simulink subsystem "ESD"  (R2020b)
settings: Solver=VariableStepAuto  StartTime=0.0  StopTime=10.0  RelTol=1e-3
undefined symbols (not defined in the file or in its folder): params
settings Model: Creator=trevor  LastModifiedBy=trevor

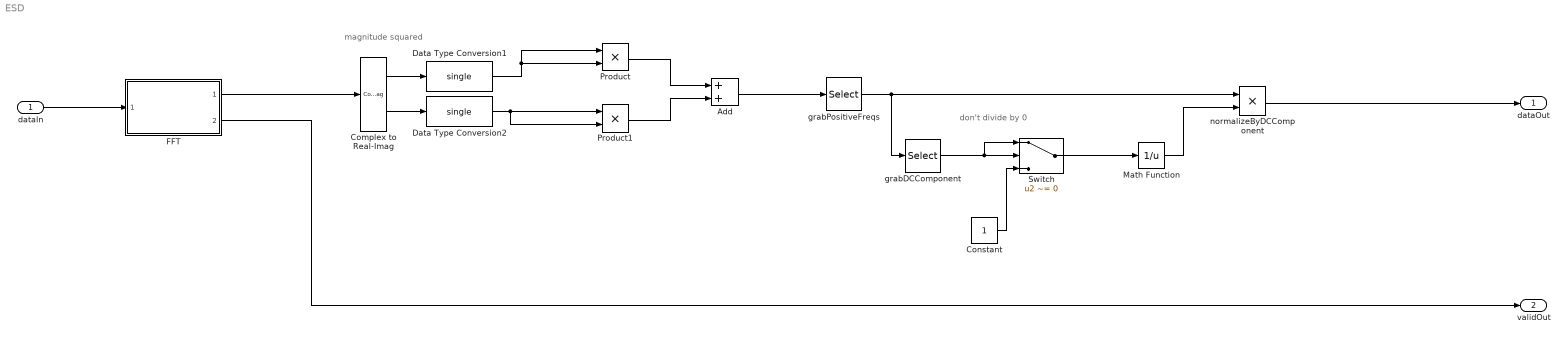
== system ESD ==
  note: don't divide by 0
  note: magnitude squared
  dataIn : Inport
  Add : Sum
  Complex to Real-Imag : ComplexToRealImag
  Constant : Constant  OutDataTypeStr=Inherit: Inherit via back propagation  SampleTime=-1
  Data Type Conversion1 : DataTypeConversion  OutDataTypeStr=single  RndMeth=Nearest
  Data Type Conversion2 : DataTypeConversion  OutDataTypeStr=single  RndMeth=Nearest
  FFT : Subsystem  ReferencedSubsystem=FFT
  Math Function : Math  Operator=reciprocal  RndMeth=Zero  SaturateOnIntegerOverflow=on  OutDataTypeStr=Inherit: Inherit via internal rule
  Product : Product
  Product1 : Product
  Switch : Switch  Criteria=u2 ~= 0
  grabDCComponent : Selector  NumberOfDimensions=2  InputPortWidth=params.FFTSize  IndexOptions=Index vector (dialog),Index vector (dialog)  Indices=[1],1  OutputSizes=1,1
  grabPositiveFreqs : Selector  NumberOfDimensions=2  InputPortWidth=params.FFTSize  IndexOptions=Index vector (dialog),Index vector (dialog)  Indices=1,[1:params.FFTSize/2]  OutputSizes=1,1
  normalizeByDCComponent : Product  Inputs=**  RndMeth=Zero  SaturateOnIntegerOverflow=on  OutDataTypeStr=Inherit: Same as first input
  dataOut : Outport
  validOut : Outport  Port=2
  wires:
  FFT/1 -> Complex to Real-Imag/1
  normalizeByDCComponent/1 -> dataOut/1
  dataIn/1 -> FFT/1
  grabPositiveFreqs/1 -> normalizeByDCComponent/1, grabDCComponent/1
  grabDCComponent/1 -> Switch/2, Switch/1
  Complex to Real-Imag/1 -> Data Type Conversion1/1
  Complex to Real-Imag/2 -> Data Type Conversion2/1
  Product1/1 -> Add/2
  Product/1 -> Add/1
  Add/1 -> grabPositiveFreqs/1
  Constant/1 -> Switch/3
  Switch/1 -> Math Function/1
  FFT/2 -> validOut/1
  Math Function/1 -> normalizeByDCComponent/2
  Data Type Conversion1/1 -> Product/1, Product/2
  Data Type Conversion2/1 -> Product1/2, Product1/1
